simulink model "Regler_Vorlage"  (R2016b)
settings: Solver=VariableStepAuto  StartTime=0.0  StopTime=10.0  RelTol=1e-3
settings Model: Creator=Fritz  LastModifiedBy=Fritz

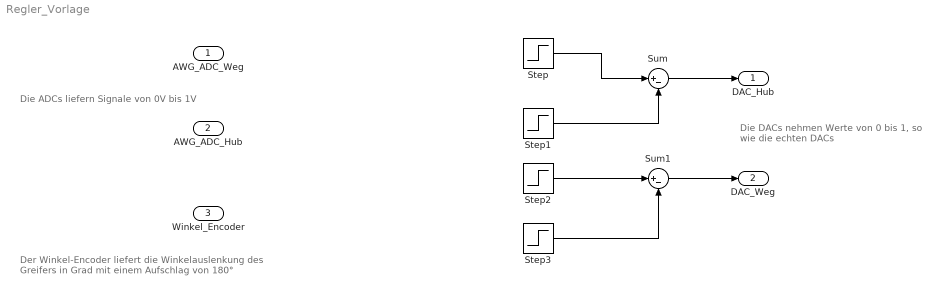
== system Regler_Vorlage ==
  note: Die DACs nehmen Werte von 0 bis 1,
      | so wie die echten DACs
  note: Der Winkel-Encoder liefert die Winkelauslenkung des
      | Greifers in Grad mit einem Aufschlag von 180°
  note: Die ADCs liefern Signale von 0V bis 1V
  AWG_ADC_Weg : Inport
  AWG_ADC_Hub : Inport  Port=2
  Winkel_Encoder : Inport  Port=3
  Step : Step  After=0.1  SampleTime=0
  Step1 : Step  Time=8  After=0.1  SampleTime=0
  Step2 : Step  After=0.1  SampleTime=0
  Step3 : Step  Time=8  After=0.1  SampleTime=0
  Sum : Sum  Inputs=|+-
  Sum1 : Sum  Inputs=|+-
  DAC_Hub : Outport
  DAC_Weg : Outport  Port=2
  wires:
  Sum/1 -> DAC_Hub/1
  Step/1 -> Sum/1
  Step1/1 -> Sum/2
  Sum1/1 -> DAC_Weg/1
  Step2/1 -> Sum1/1
  Step3/1 -> Sum1/2
